simulink model "scenario2"  (R2020a)
settings: Solver=FixedStepAuto  StartTime=0.0  StopTime=20  MaxStep=0.01  RelTol=1e-4  EnableMultiTasking=on
undefined symbols (not defined in the file or in its folder): sigbuilder_block
libraries: fuzblock x1
settings Model: Creator=root  LastModifiedBy=Leonidas
settings DataIOCC: LimitDataPoints=on  SaveOutput=off  SaveTime=off  ReturnWorkspaceOutputs=off
settings OptimizationCC: ExpressionDepthLimit=2147483647  LifeSpan=1
settings DebuggingCC: UnderspecifiedInitializationDetection=Classic  MergeDetectMultiDrivingBlocksExec=none  FcnCallInpInsideContextMsg=warning  AllowSymbolicDim=off  StateNameClashWarn=warning  SFUnexpectedBacktrackingDiag=warning  SFNoUnconditionalDefaultTransitionDiag=warning  SFExecutionAtInitializationDiag=none  ArithmeticOperatorsInVariantConditions=warning
settings SFSimCC: SimUseLocalCustomCode=off  CustomCodeUndefinedFunction=UseInterfaceOnly
settings RTWCC: RTWUseLocalCustomCode=off
settings CodeAppCC: StateflowObjectComments=on
settings GRTTargetCC: TargetLangStandard=C89/C90 (ANSI)  CombineOutputUpdateFcns=off  GRTInterface=on

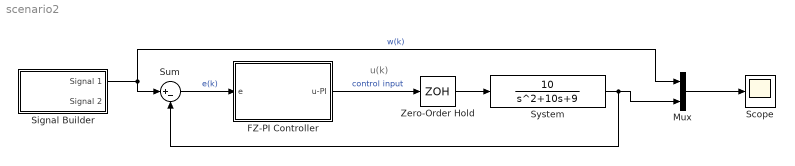
== system scenario2 ==
  note: u(k)
  FZ-PI Controller : Subsystem
  Mux : Mux  Inputs=2
  Scope : Scope
  Signal Builder : Subsystem  Tag=STV Subsys  LoadFcn=sigbuilder_block('load');  StartFcn=sigbuilder_block('start');  StopFcn=sigbuilder_block('stop');  ClipboardFcn=sigbuilder_block('clipboard');  mask(Sigbuilder block){tuvar=[0:10]}
      mask help: Simulink:masks:SigbuilderBlock_MD
      mask init:
      | if ~strcmp(get_param(bdroot(gcbh),'SimulationStatus'),'stopped') tuvar = sigbuilder_block('maskInit'); end
      settings: CopyFcn=sigbuilder_block('copy');  DeleteFcn=sigbuilder_block('delete');  ModelCloseFcn=sigbuilder_block('modelClose');  PreSaveFcn=sigbuilder_block('preSave');  PauseFcn=sigbuilder_block('pause');  ContinueFcn=sigbuilder_block('continue');  NameChangeFcn=sigbuilder_block('namechange');  OpenFcn=sigbuilder_block('open',[6 30 1428 681.75 ]);  CloseFcn=sigbuilder_block('close');
      mask Display: plot(0, 0, 100, 100,[2, 2, 32, 32, 2], [68, 8, 8, 68, 68],[32, 2], [38, 38], [32, 19, 2],[53, 60, 44], [32, 17, 17, 2],[16, 16, 31, 31]);txt = getActiveGroup(gcbh);text(2, 100, txt,'verticalAlignment', 'top');
  Sum : Sum  Inputs=|+-
  System : TransferFcn  Numerator=[10]  Denominator=[1 10 9]
  Zero-Order Hold : ZeroOrderHold  SampleTime=0.01
  wires:
  Sum/1 -> FZ-PI Controller/1(e)  "e(k)"
  FZ-PI Controller/1(u-PI) -> Zero-Order Hold/1  "control input"
  Zero-Order Hold/1 -> System/1
  System/1 -> Sum/2, Mux/2
  Mux/1 -> Scope/1
  Signal Builder/1(Signal 1) -> Sum/1, Mux/1  "w(k)"

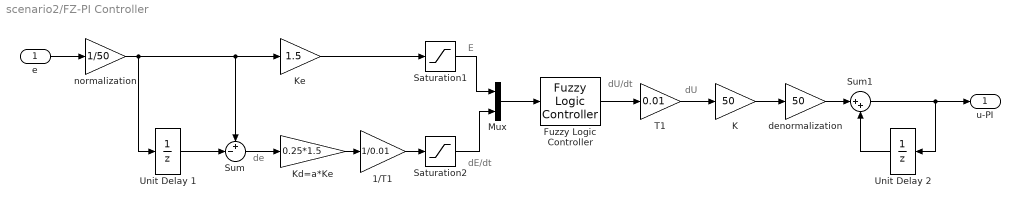
== system scenario2/FZ-PI Controller ==
  note: E
  note: de
  note: dE/dt
  note: dU/dt
  note: dU
  e : Inport
  1/T1 : Gain  Gain=1/0.01
  Fuzzy Logic Controller : fuzblock/Fuzzy Logic  Controller  FIS='satellite.fis_obj'  OutputSampleNumber=101  DataType=double  FuzzifiedInputs=off  RuleFiringStrengths=off  RuleOutputs=off  AggregatedOutputs=off  SimulateUsing=Interpreted execution  OutOfRangeInputValueMessage=warning  NoRuleFiredMessage=warning  EmptyOutputFuzzySetMessage=warning
  K : Gain  Gain=50
  Kd=a*Ke : Gain  Gain=0.25*1.5
  Mux : Mux  Inputs=2
  Saturation1 : Saturate  UpperLimit=1  LowerLimit=-1
  Saturation2 : Saturate  UpperLimit=1  LowerLimit=-1
  Sum : Sum  Inputs=+-|
  Sum1 : Sum  Inputs=|++
  "T1 " : Gain  Gain=0.01
  Unit Delay 1 : UnitDelay  SampleTime=0.01  HasFrameUpgradeWarning=on
  Unit Delay 2 : UnitDelay  SampleTime=0.01  HasFrameUpgradeWarning=on
  denormalization : Gain  Gain=50
  normalization : Gain  Gain=1/50
  Κe : Gain  Gain=1.5
  u-PI : Outport  VectorParamsAs1DForOutWhenUnconnected=off
  wires:
  e/1 -> normalization/1
  normalization/1 -> Unit Delay 1/1, Sum/1, Κe/1
  Unit Delay 1/1 -> Sum/2
  Sum/1 -> Kd=a*Ke/1
  Kd=a*Ke/1 -> 1/T1/1
  Κe/1 -> Saturation1/1
  1/T1/1 -> Saturation2/1
  Saturation1/1 -> Mux/1
  Saturation2/1 -> Mux/2
  Mux/1 -> Fuzzy Logic Controller/1
  Fuzzy Logic Controller/1 -> "T1 "/1
  "T1 "/1 -> K/1
  K/1 -> denormalization/1
  denormalization/1 -> Sum1/1
  Sum1/1 -> u-PI/1, Unit Delay 2/1
  Unit Delay 2/1 -> Sum1/2

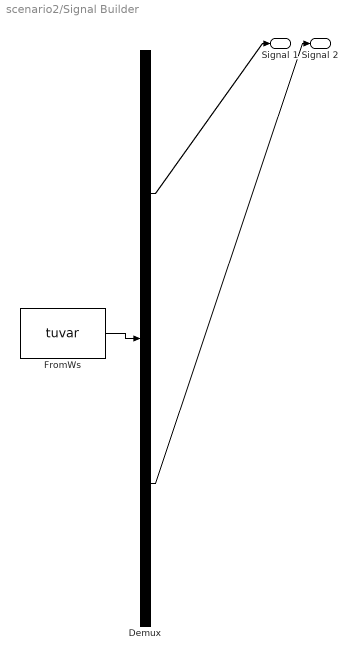
== system scenario2/Signal Builder ==
  Demux : Demux  Tag=STV Demux  Outputs=2
      settings: DisplayOption=none
  FromWs : FromWorkspace  Tag=STV FromWs  VariableName=tuvar
      SigBuilderData=|
      | common.afterFinalStr = 'Extrapolate'
      | common.sampleTime = 0
      | dataSet.timeRange = [0 16]
      | dataSet.name = 'Group 1'
      | sbobj.Groups.Name = 'Group 1'
      | sbobj.Groups.Signals(1).Name = 'Signal 1'
      | sbobj.Groups.Signals(1).XData = [0 4 4 8 8 16]
      | sbobj.Groups.Signals(1).YData = [60 60 20 20 40 40]
      | sbobj.Groups.Signals(2).Name = 'Signal 2'
      | sbobj.Groups.Signals(2).XData = [0 5 8 16]
      | sbobj.Groups.Signals(2).YData = [0 60 60 0]
      | sbobj.Groups.TimeRange = [0 16]
  Signal 1 : Outport  Tag=STV Outport  VectorParamsAs1DForOutWhenUnconnected=off
  Signal 2 : Outport  Tag=STV Outport  Port=2  VectorParamsAs1DForOutWhenUnconnected=off
  wires:
  FromWs/1 -> Demux/1
  Demux/1 -> Signal 1/1
  Demux/2 -> Signal 2/1
